simulink model "IntegradorPorTrapecios"  (R2023b)
settings: Solver=VariableStepAuto  StartTime=0.0  StopTime=10.0  RelTol=1e-3
values from neighbouring files (symbols this model uses):
  T_sdis = 6*10^-5    (= 6e-05)    [varLC.m]
settings Model: Creator=gonza  LastModifiedBy=tomas

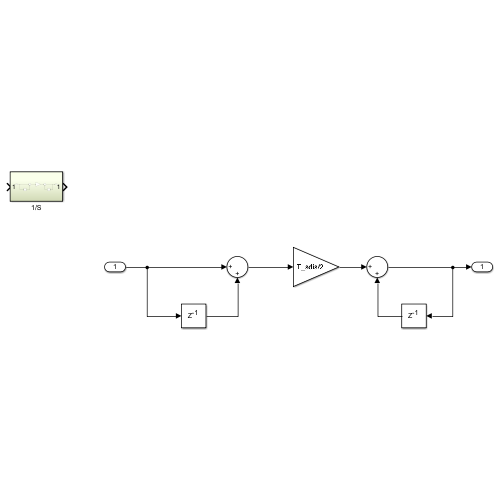
[thumbnail: Simulink's stored preview of the top-level diagram]
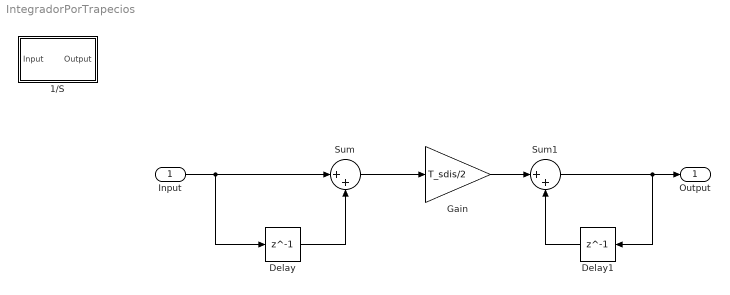
== system IntegradorPorTrapecios ==
  Input : Inport
  1/S : Subsystem
  Delay : Delay  DelayLength=1
  Delay1 : Delay  DelayLength=1
  Gain : Gain  Gain=T_sdis/2
  Sum : Sum  Inputs=|++
  Sum1 : Sum  Inputs=|++
  Output : Outport
  wires:
  Input/1 -> Delay/1, Sum/1
  Delay/1 -> Sum/2
  Sum/1 -> Gain/1
  Gain/1 -> Sum1/1
  Delay1/1 -> Sum1/2
  Sum1/1 -> Delay1/1, Output/1

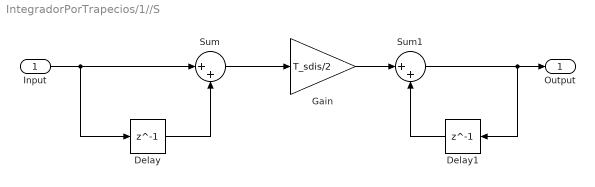
== system IntegradorPorTrapecios/1//S ==
  Input : Inport
  Delay : Delay  DelayLength=1
  Delay1 : Delay  DelayLength=1
  Gain : Gain  Gain=T_sdis/2
  Sum : Sum  Inputs=|++
  Sum1 : Sum  Inputs=|++
  Output : Outport
  wires:
  Delay/1 -> Sum/2
  Sum/1 -> Gain/1
  Gain/1 -> Sum1/1
  Sum1/1 -> Delay1/1, Output/1
  Delay1/1 -> Sum1/2
  Input/1 -> Delay/1, Sum/1
